simulink model "loopShapingSubsystem"  (Simulink 8.5)
settings: Solver=ode45  StartTime=0.0  StopTime=10  RelTol=1e-3
values from neighbouring files (symbols this model uses):
  A = [0 1; 0 -c/m]    [Untitled2.m]    (also in define_consts.m; loadProperties.m; t.mat = [0  1; 0  -0.025]; test.m)
  B = [0;1/m]    [Untitled2.m]    (also in define_consts.m; loadProperties.m; t.mat = [0 0.1]; test.m = [0 0;1/m 0])
  C = [1 0]    [Untitled2.m]    (also in deadline4.m = tf([4, 1],[0, 2]); define_consts.m; loadProperties.m; t.mat)
  C_Gain = C_Gains(i)    [LoopShapingGain.m]    (also in LoopShapingLeadCompensator.m = 1)
  cutoff = cutoffs(i)    [LoopShapingFilter.m]    (also in LoopShapingFilterNoisy.m; LoopShapingFinal.m = 100; LoopShapingFinalCrossover.m = 100; LoopShapingNoise.m = 100)
  s = ss(A,B,C,D)    [LoopShapingFinal.m]    (also in LoopShapingFinalCrossover.m; LoopShapingNoise.m; LoopShapingTest.m; LoopsShapingCrossover.m)
  wp = Ratio(i) * wz    [LoopShapingLeadCompensator.m]
  wz = 1    [LoopShapingLeadCompensator.m]
libraries: slctrlblks x1
settings Model: Creator=Adrien  LastModifiedBy=Adrien
settings DataIOCC: SignalLoggingSaveFormat=Dataset
settings OptimizationCC: ExpressionDepthLimit=128
settings DebuggingCC: UnderspecifiedInitializationDetection=Simplified  MergeDetectMultiDrivingBlocksExec=error  FcnCallInpInsideContextMsg=EnableAllAsError  StateNameClashWarn=none
settings GRTTargetCC: CombineOutputUpdateFcns=on  GRTInterface=off

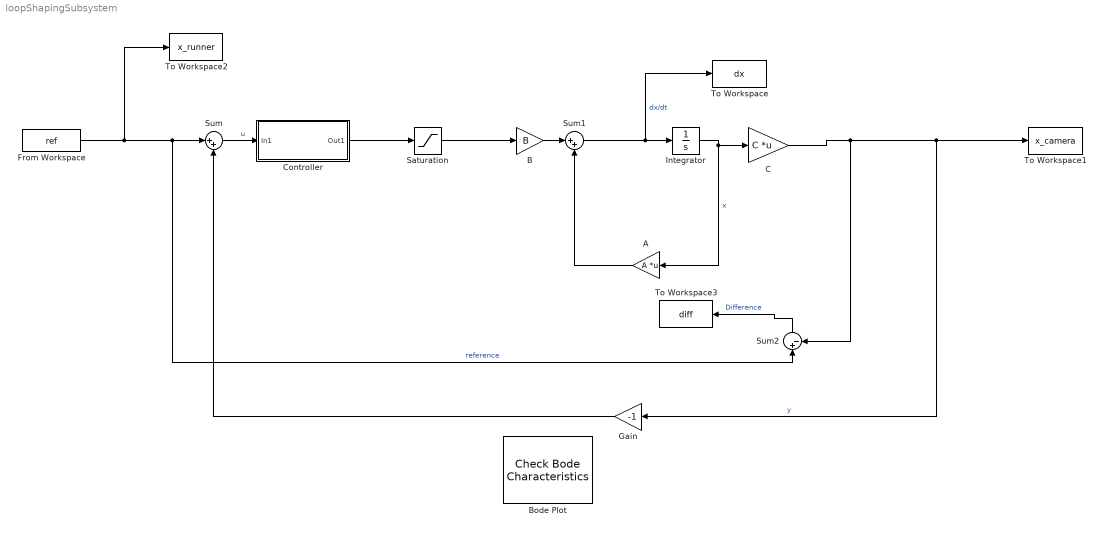
== system loopShapingSubsystem ==
  A : Gain  Gain=A  Multiplication=Matrix(K*u) (u vector)
  "B  " : Gain  Gain=B
  Bode Plot : slctrlblks/Model Verification/Check Bode  Characteristics  InstantiateOnLoad=on  SaveOperatingPoints=off  LinearizationIOs={'/C ', 1, 'out', 'on', '';'/Sum', 1, 'in', 'off', ''}  LinearizeAt=SnapshotTimes  SnapshotTimes=[0]  TriggerType=rising  SampleTime=auto  RateConversionMethod=zoh  PreWarpFreq=10  UseExactDelayModel=off  UseFullBlockNameLabels=off  UseBusSignalLabels=off  enabled=on  stopWhenAssertionFail=off  export=off  ViewDlgPos=[100 200 510 390]  OpenViewOnLoad=off  LaunchViewOnOpen=off  FrequencyUnits=rad/s  MagnitudeUnits=dB  PhaseUnits=deg  TimeUnits=seconds  EnableUpperBound=off  UpperBoundFrequencies=[]  UpperBoundMagnitudes=[]  EnableLowerBound=off  LowerBoundFrequencies=[]  LowerBoundMagnitudes=[]
      settings: SaveToWorkspace=on
  "C " : Gain  Gain=C  Multiplication=Matrix(K*u) (u vector)
  "Controller " : Subsystem
  From Workspace : FromWorkspace  VariableName=ref  SampleTime=step  Interpolate=off  OutputAfterFinalValue=Holding final value
  "Gain " : Gain  Gain=-1
  Integrator : Integrator  InitialCondition=[0 0]
  Saturation : Saturate  UpperLimit=70  LowerLimit=-70
  Sum : Sum  Inputs=|++
  Sum1 : Sum  Inputs=|++
  Sum2 : Sum  Inputs=|+-
  To Workspace : ToWorkspace  VariableName=dx  SaveFormat=Timeseries  SampleTime=-1
  To Workspace1 : ToWorkspace  VariableName=x_camera  SaveFormat=Timeseries  SampleTime=-1
  To Workspace2 : ToWorkspace  VariableName=x_runner  SaveFormat=Timeseries  SampleTime=-1
  To Workspace3 : ToWorkspace  VariableName=diff  SaveFormat=Timeseries  SampleTime=-1
  wires:
  Integrator/1 -> A/1, "C "/1  "x"
  "B  "/1 -> Sum1/1
  A/1 -> Sum1/2
  From Workspace/1 -> To Workspace2/1, Sum/1, Sum2/1  "reference"
  "C "/1 -> Sum2/2, "Gain "/1, To Workspace1/1  "y"
  Sum1/1 -> To Workspace/1, Integrator/1  "dx/dt"
  Sum2/1 -> To Workspace3/1  "Difference"
  Saturation/1 -> "B  "/1
  "Gain "/1 -> Sum/2
  Sum/1 -> "Controller "/1(In1)  "u"
  "Controller "/1(Out1) -> Saturation/1

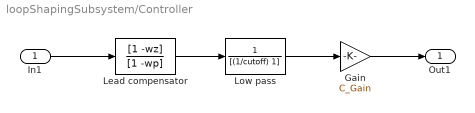
== system loopShapingSubsystem/Controller  ==
  In1 : Inport
  Gain : Gain  Gain=C_Gain
  "Lead compensator " : TransferFcn  Numerator=[1 -wz]  Denominator=[1 -wp]
  "Low pass " : TransferFcn  Denominator=[(1/cutoff) 1]
  Out1 : Outport
  wires:
  In1/1 -> "Lead compensator "/1
  Gain/1 -> Out1/1
  "Lead compensator "/1 -> "Low pass "/1
  "Low pass "/1 -> Gain/1
